simulink model "lift"  (R2020b)
settings: Solver=VariableStepAuto  StartTime=0.0  StopTime=10.0  RelTol=1e-3
settings Model: Creator=priyaD  LastModifiedBy=priyaD

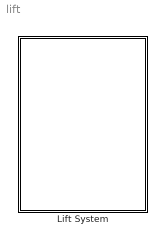
== system lift ==
  Lift System : Stateflow chart  TreatAsAtomicUnit=on

== stateflow chart lift/Lift System ==
  state enqueue(hall_call_floor) [function]
    (default) -> (junction 12)
    (junction 12) -> (junction 15) [order 1] : [hall_call_status [hall_call_floor] ~= 0]
    (junction 12) -> (junction 17) [order 2] : {i=0;}
    (junction 17) -> (junction 19) [order 1] : [hall_call_queue[i] == hall_call_floor]
    (junction 17) -> (junction 17) [order 2]
    (junction 17) -> (junction 28) [order 3] : [hall_call_queue[i] > 0 && i<NUM_FLOOR]{i = i + 1;}
    (junction 28) -> (junction 29) [order 1] : [i>=NUM_FLOOR]
    (junction 28) -> (junction 31) [order 2] : {hall_call_queue[i] = hall_call_floor;}
  state register(hall_call_floor) [function]
    (default) -> (junction 4) : {enqueue(hall_call_floor);
        | hall_call_status [hall_call_floor]=1;}
  data: hall_call_floor function_input; hall_call_floor function_input
